simulink model "Explorer1632_dsPIC33EP512MU810_UART_Terminal_R2015b"  (R2015b)
settings: Solver=FixedStepDiscrete  StartTime=0.0  StopTime=inf  FixedStep=0.01  RelTol=1e-3
undefined symbols (not defined in the file): A0, D0, DiscIntNeverNeededParam, F4, F5, Max, ms, P100, P101, P16, P64, Pin, Resol, us
libraries: MCHP_Blockset x40, simulink x11
(part 2 of 2)

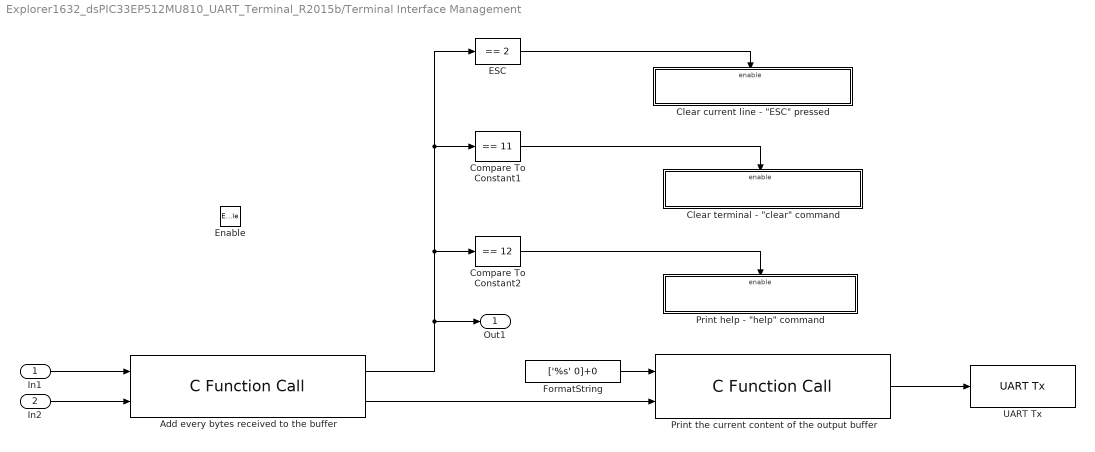
== system Explorer1632_dsPIC33EP512MU810_UART_Terminal_R2015b/Terminal Interface Management ==
  In1 : Inport
  In2 : Inport  Port=2
  Enable : EnablePort
  Add every bytes received to the buffer : MCHP_Blockset/User Functions/C Function Call  Priority=0  ParseFilesChkbx=off  ListFunctions1=Custom Function  Function1=unsigned char addToBuffer( unsigned char outputBuffer[100], unsigned char *rxBuffer, unsigned int rxCnt)  AddHeaderDeclaration=off  Function1Type=when block is updated (default)  Fct1BlockIn=rxBuffer, rxCnt  FctReturnBlockOut=on  Fct1BlockOut=outputBuffer  DataCollected=0  ORDERING=None  SampleTime=-1  S_INPUT="[2  5]"  S_INPUT_Size="[-1  0  0  0  0  0  0  0  0  0  0  0  0  0  0  0  0  0  0  0]"  S_OUTPUT=[2]  S_OUTPUT_Size="[1  17   0   0   0   0   0   0   0   0]"  S_ListCustomDatatype=S.S_ListCustomDatatype={};  MCHP_CRC=1191397  MCHP_MASTERLINK=Explorer1632_dsPIC33EP512MU810_UART_Terminal_R2015b/Explorer16//32 - dsPIC33EP512MU810/Microchip Master  PinDigitalInput=[]  PinDigitalOutput=[]  PinAnalogInput=[]
  "Clear current line - \"ESC\" pressed" : Subsystem  Priority=1  TreatAsAtomicUnit=on
  "Clear terminal - \"clear\" command" : Subsystem  Priority=100
  Compare To Constant1 : simulink/Logic and Bit Operations/Compare To Constant  relop===  const=11  OutDataTypeStr=uint8
  Compare To Constant2 : simulink/Logic and Bit Operations/Compare To Constant  relop===  const=12  OutDataTypeStr=uint8
  ESC : simulink/Logic and Bit Operations/Compare To Constant  relop===  const=2  OutDataTypeStr=uint8
  "FormatString " : Constant  Priority=15  Value=['%s' 0]+0  OutDataTypeStr=uint8  LockScale=on
  "Print help - \"help\" command" : Subsystem  Priority=99
  Print the current content of the output buffer : MCHP_Blockset/User Functions/C Function Call  Priority=16  ParseFilesChkbx=off  ListFunctions1=Custom Function  Function1=void sprintf(unsigned char outputBuffer[100], const unsigned char* formatString, unsigned char* rxBuffer)  AddHeaderDeclaration=off  Function1Type=when block is updated (default)  Fct1BlockIn=formatString , rxBuffer  FctReturnBlockOut=off  Fct1BlockOut=outputBuffer  DataCollected=0  ORDERING=None  SampleTime=-1  S_INPUT="[2  5]"  S_INPUT_Size="[-1  0  0  0  0  0  0  0  0  0  0  0  0  0  0  0  0  0  0  0]"  S_OUTPUT=[2]  S_OUTPUT_Size="[1  17   0   0   0   0   0   0   0   0]"  S_ListCustomDatatype=S.S_ListCustomDatatype={};  MCHP_CRC=1218869  MCHP_MASTERLINK=Explorer1632_dsPIC33EP512MU810_UART_Terminal_R2015b/Explorer16//32 - dsPIC33EP512MU810/Microchip Master  PinDigitalInput=[]  PinDigitalOutput=[]  PinAnalogInput=[]
  UART Tx : MCHP_Blockset/BUS UART/UART Tx  Priority=17  UART_REF=1  ORDERING=None  AllOrNothing=off  SampleTime=-1  MCHP_MASTERLINK=Explorer1632_dsPIC33EP512MU810_UART_Terminal_R2015b/Explorer16//32 - dsPIC33EP512MU810/Microchip Master  NSend_Input=off  UART_String=on  NSend_Output=off
  Out1 : Outport
  wires:
  In1/1 -> Add every bytes received to the buffer/1
  In2/1 -> Add every bytes received to the buffer/2
  "FormatString "/1 -> Print the current content of the output buffer/1
  Print the current content of the output buffer/1 -> UART Tx/1
  Add every bytes received to the buffer/2 -> Print the current content of the output buffer/2
  Add every bytes received to the buffer/1 -> Compare To Constant2/1, ESC/1, Compare To Constant1/1, Out1/1
  Compare To Constant1/1 -> "Clear terminal - \"clear\" command"/Enable
  Compare To Constant2/1 -> "Print help - \"help\" command"/Enable
  ESC/1 -> "Clear current line - \"ESC\" pressed"/Enable

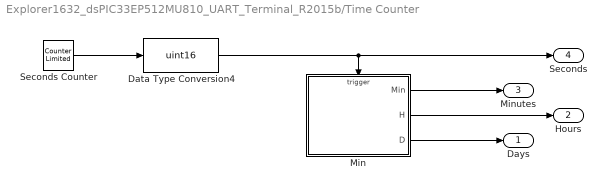
== system Explorer1632_dsPIC33EP512MU810_UART_Terminal_R2015b/Time Counter ==
  Data Type Conversion4 : DataTypeConversion  OutDataTypeStr=uint16  ConvertRealWorld=Stored Integer (SI)
  Min : Subsystem
  Seconds Counter : simulink/Sources/Counter Limited  uplimit=59  tsamp=1
  Days : Outport
  Hours : Outport  Port=2
  Minutes : Outport  Port=3
  Seconds : Outport  Port=4
  wires:
  Data Type Conversion4/1 -> Min/Trigger, Seconds/1
  Seconds Counter/1 -> Data Type Conversion4/1
  Min/1(Min) -> Minutes/1
  Min/2(H) -> Hours/1
  Min/3(D) -> Days/1

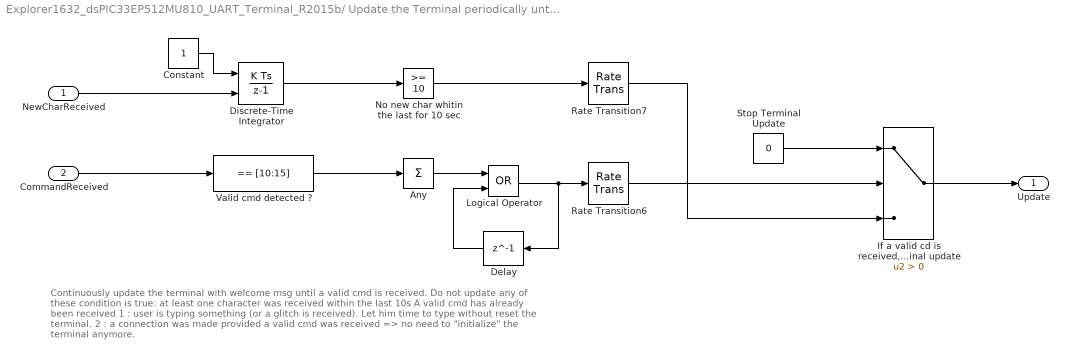
== system Explorer1632_dsPIC33EP512MU810_UART_Terminal_R2015b/ Update the Terminal periodically until a connection is detected /Periodic update until a valid cmd is received ==
  note: Continuously update the terminal with welcome msg until a valid cmd is received.
      |
      | Do not update any of these condition is true:
      | at least one character was received within the last 10s
      | A valid cmd has already been received
      |
      | 1 : user is typing something (or a glitch is received). Let him time to type without reset the terminal.
      | 2 : a connection was made provided a valid cmd was received => no need to "initialize" the terminal anymore.
  NewCharReceived : Inport
  CommandReceived : Inport  Port=2
  Any : Sum  Inputs=+
  Constant : Constant  OutDataTypeStr=uint16  SampleTime=.01
  Delay : Delay  DelayLength=1  InitialCondition=0
  Discrete-Time Integrator : DiscreteIntegrator  gainval=1  ExternalReset=level  InitialConditionSetting=State (most efficient)  SampleTime=-1  OutMax=[10]  OutDataTypeStr=fixdt(0,16)  SaturateOnIntegerOverflow=on  ICPrevOutput=DiscIntNeverNeededParam  ICPrevScaledInput=DiscIntNeverNeededParam
  "If a valid cd is received, then disable the trigger for terminal update" : Switch  Criteria=u2 > Threshold
  Logical Operator : Logic  Operator=OR  AllPortsSameDT=off  OutDataTypeStr=boolean
  No new char whitin the last for 10 sec : simulink/Logic and Bit Operations/Compare To Constant  relop=>=  const=10  OutDataTypeStr=boolean
  Rate Transition6 : RateTransition  Integrity=off  Deterministic=off  OutPortSampleTime=2
  Rate Transition7 : RateTransition  Integrity=off  Deterministic=off  OutPortSampleTime=2
  Stop Terminal Update : Constant  Value=0  OutDataTypeStr=uint16  SampleTime=-1
  Valid cmd detected ? : simulink/Logic and Bit Operations/Compare To Constant  relop===  const=[10:15]  OutDataTypeStr=boolean
  Update : Outport
  wires:
  NewCharReceived/1 -> Discrete-Time Integrator/2
  CommandReceived/1 -> Valid cmd detected ?/1
  Constant/1 -> Discrete-Time Integrator/1
  Valid cmd detected ?/1 -> Any/1
  Logical Operator/1 -> Delay/1, Rate Transition6/1
  Delay/1 -> Logical Operator/2
  Any/1 -> Logical Operator/1
  No new char whitin the last for 10 sec/1 -> Rate Transition7/1
  Discrete-Time Integrator/1 -> No new char whitin the last for 10 sec/1
  "If a valid cd is received, then disable the trigger for terminal update"/1 -> Update/1
  Stop Terminal Update/1 -> "If a valid cd is received, then disable the trigger for terminal update"/1
  Rate Transition6/1 -> "If a valid cd is received, then disable the trigger for terminal update"/2
  Rate Transition7/1 -> "If a valid cd is received, then disable the trigger for terminal update"/3

== system Explorer1632_dsPIC33EP512MU810_UART_Terminal_R2015b/ Update the Terminal periodically until a connection is detected /Periodic update until first character is received ==
  NewCharReceived : Inport
  Any char received? : simulink/Logic and Bit Operations/Compare To Constant  relop=>=  const=1  OutDataTypeStr=boolean
  Delay1 : Delay  DelayLength=1  InitialCondition=0
  Logical Operator : Logic  Operator=NOT  AllPortsSameDT=off  OutDataTypeStr=boolean
  Logical Operator1 : Logic  Operator=OR  AllPortsSameDT=off  OutDataTypeStr=boolean
  Rate Transition3 : RateTransition  Integrity=off  Deterministic=off  OutPortSampleTime=2
  Out1 : Outport
  wires:
  Any char received?/1 -> Logical Operator1/1
  NewCharReceived/1 -> Any char received?/1
  Rate Transition3/1 -> Out1/1
  Logical Operator/1 -> Rate Transition3/1
  Delay1/1 -> Logical Operator1/2
  Logical Operator1/1 -> Logical Operator/1, Delay1/1

== system Explorer1632_dsPIC33EP512MU810_UART_Terminal_R2015b/ Update the Terminal periodically until a connection is detected /Terminal Initialization ==
  note: Re-initialize the terminal and display the main menu every 2 second until a valid cmd is received. This allows initializing hot plugged terminal.
  note: => command to r eset the terminal to initial state:
      | Go home and then set green color for text
  Enable : EnablePort
  Constant7 : Constant  Priority=0  Value="[27 99  0]+0"  OutDataTypeStr=int8  LockScale=on
  "Print help - \"help\" command" : Subsystem  Priority=99
  UART Tx1 : MCHP_Blockset/BUS UART/UART Tx  UART_REF=1  ORDERING=None  AllOrNothing=off  SampleTime=-1  MCHP_MASTERLINK=Explorer1632_dsPIC33EP512MU810_UART_Terminal_R2015b/Explorer16//32 - dsPIC33EP512MU810/Microchip Master  NSend_Input=off  UART_String=on  NSend_Output=off
  wires:
  Constant7/1 -> UART Tx1/1

== system Explorer1632_dsPIC33EP512MU810_UART_Terminal_R2015b/Data Collector/Temperature Calibration  ==
  Temp raw : Inport
  "100 deg / Volt " : Gain  Gain=3.3/(2^16) * 100  OutDataTypeStr=single
  Calibration Offset 500 mv at 0 deg : Constant  Value=50  OutDataTypeStr=Inherit: Inherit via back propagation  SampleTime=-1
  Sum2 : Sum  Inputs=|+-  OutDataTypeStr=Inherit: Same as first input
  Temp degC : Outport
  wires:
  Temp raw/1 -> "100 deg / Volt "/1
  "100 deg / Volt "/1 -> Sum2/1
  Calibration Offset 500 mv at 0 deg/1 -> Sum2/2
  Sum2/1 -> Temp degC/1  "deg"

== system Explorer1632_dsPIC33EP512MU810_UART_Terminal_R2015b/Explorer16//32 - dsPIC33EP512MU810/Open board Documentation ==

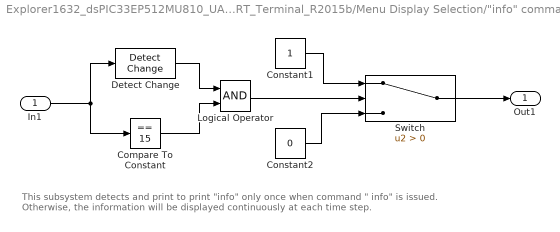
== system Explorer1632_dsPIC33EP512MU810_UART_Terminal_R2015b/Menu Display Selection/"info" command detection ==
  note: This subsystem detects and print to print "info" only once when command " info" is issued. Otherwise, the information will be displayed continuously at each time step.
  In1 : Inport
  Compare To Constant : simulink/Logic and Bit Operations/Compare To Constant  relop===  const=15  OutDataTypeStr=uint8
  Constant1 : Constant  OutDataTypeStr=uint16
  Constant2 : Constant  Value=0  OutDataTypeStr=uint16
  Detect Change : simulink/Logic and Bit Operations/Detect Change  vinit=0  OutDataTypeStr=boolean
  Logical Operator : Logic  AllPortsSameDT=off  OutDataTypeStr=boolean
  Switch : Switch  Criteria=u2 > Threshold
  Out1 : Outport
  wires:
  Constant2/1 -> Switch/3
  Constant1/1 -> Switch/1
  Switch/1 -> Out1/1
  Compare To Constant/1 -> Logical Operator/2
  Logical Operator/1 -> Switch/2
  Detect Change/1 -> Logical Operator/1
  In1/1 -> Detect Change/1, Compare To Constant/1

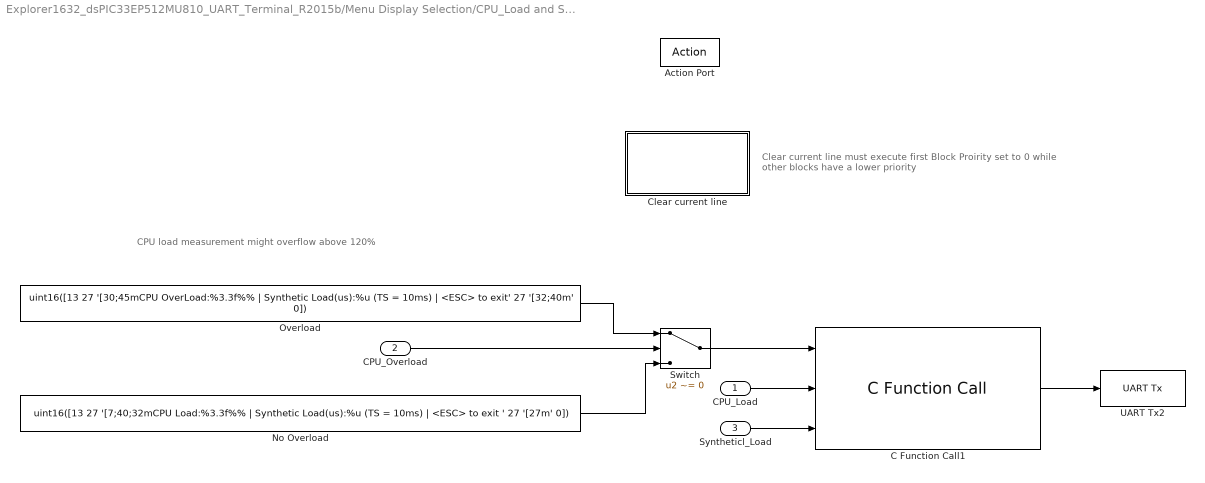
== system Explorer1632_dsPIC33EP512MU810_UART_Terminal_R2015b/Menu Display Selection/CPU_Load and Synthetic_Load ==
  note: Clear current line must execute first
      | Block Proirity set to 0 while other blocks have a lower priority
  note: CPU load measurement might overflow above 120%
  CPU_Load : Inport
  CPU_Overload : Inport  Port=2
  Syntheticl_Load : Inport  Port=3
  Action Port : ActionPort  ActionType=case
  C Function Call1 : MCHP_Blockset/User Functions/C Function Call  Priority=20  ParseFilesChkbx=off  ListFunctions1=Custom Function  Function1=void sprintf(char outputBuffer[100], const char* formatString, float arg1, unsigned int arg2)  AddHeaderDeclaration=off  Function1Type=when block is updated (default)  Fct1BlockIn=formatString , arg1, arg2  FctReturnBlockOut=off  Fct1BlockOut=outputBuffer  DataCollected=0  ORDERING=None  SampleTime=-1  S_INPUT="[2  5]"  S_INPUT_Size="[-1  0  0  0  0  0  0  0  0  0  0  0  0  0  0  0  0  0  0  0]"  S_OUTPUT=[2]  S_OUTPUT_Size="[1  17   0   0   0   0   0   0   0   0]"  S_ListCustomDatatype=S.S_ListCustomDatatype={};  MCHP_CRC=1179584  MCHP_MASTERLINK=Explorer1632_dsPIC33EP512MU810_UART_Terminal_R2015b/Explorer16//32 - dsPIC33EP512MU810/Microchip Master  PinDigitalInput=[]  PinDigitalOutput=[]  PinAnalogInput=[]
  Clear current line : Subsystem  Priority=0  TreatAsAtomicUnit=on
  No Overload : Constant  Value="uint16([13 27 '[7;40;32mCPU Load:%3.3f%% |  Synthetic Load(us):%u (TS = 10ms) | <ESC> to exit     ' 27 '[27m'  0])"  OutDataTypeStr=int8  LockScale=on
  Overload : Constant  Value="uint16([13 27 '[30;45mCPU OverLoad:%3.3f%% |  Synthetic Load(us):%u (TS = 10ms) | <ESC> to exit' 27 '[32;40m'  0])"  OutDataTypeStr=int8  LockScale=on
  Switch : Switch  Criteria=u2 ~= 0
  UART Tx2 : MCHP_Blockset/BUS UART/UART Tx  UART_REF=1  ORDERING=None  AllOrNothing=off  SampleTime=-1  MCHP_MASTERLINK=Explorer1632_dsPIC33EP512MU810_UART_Terminal_R2015b/Explorer16//32 - dsPIC33EP512MU810/Microchip Master  NSend_Input=off  UART_String=on  NSend_Output=off
  wires:
  C Function Call1/1 -> UART Tx2/1
  CPU_Load/1 -> C Function Call1/2
  Syntheticl_Load/1 -> C Function Call1/3
  CPU_Overload/1 -> Switch/2
  Switch/1 -> C Function Call1/1
  No Overload/1 -> Switch/3
  Overload/1 -> Switch/1

== system Explorer1632_dsPIC33EP512MU810_UART_Terminal_R2015b/Menu Display Selection/Info ==
  In1 : Inport
  Action Port : ActionPort  ActionType=case
  "Print \"info\"" : Subsystem
  wires:
  In1/1 -> "Print \"info\""/Enable

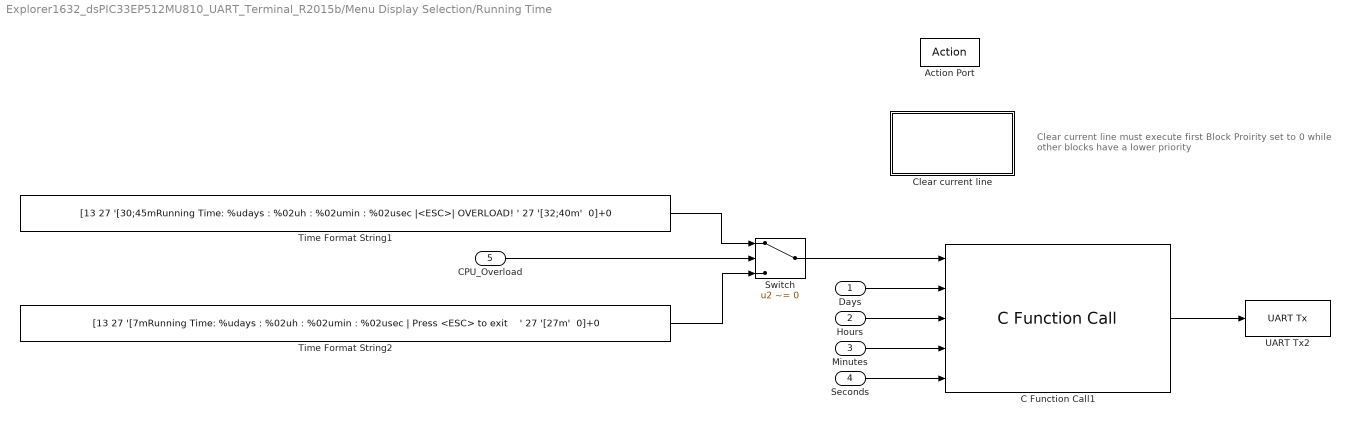
== system Explorer1632_dsPIC33EP512MU810_UART_Terminal_R2015b/Menu Display Selection/Running Time ==
  note: Clear current line must execute first
      | Block Proirity set to 0 while other blocks have a lower priority
  Days : Inport
  Hours : Inport  Port=2
  Minutes : Inport  Port=3
  Seconds : Inport  Port=4
  CPU_Overload : Inport  Port=5
  Action Port : ActionPort  ActionType=case
  C Function Call1 : MCHP_Blockset/User Functions/C Function Call  ParseFilesChkbx=off  ListFunctions1=Custom Function  Function1=void sprintf(char outputBuffer[100], const char* formatString, unsigned int days,unsigned int hours,unsigned int minutes,unsigned int seconds)  AddHeaderDeclaration=off  Function1Type=when block is updated (default)  Fct1BlockIn=formatString, days, , hours, minutes, seconds  FctReturnBlockOut=off  Fct1BlockOut=outputBuffer  DataCollected=0  ORDERING=None  SampleTime=-1  S_INPUT="[2  5]"  S_INPUT_Size="[-1  0  0  0  0  0  0  0  0  0  0  0  0  0  0  0  0  0  0  0]"  S_OUTPUT=[2]  S_OUTPUT_Size="[1  17   0   0   0   0   0   0   0   0]"  S_ListCustomDatatype=S.S_ListCustomDatatype={};  MCHP_CRC=1463372  MCHP_MASTERLINK=Explorer1632_dsPIC33EP512MU810_UART_Terminal_R2015b/Explorer16//32 - dsPIC33EP512MU810/Microchip Master  PinDigitalInput=[]  PinDigitalOutput=[]  PinAnalogInput=[]
  Clear current line : Subsystem  Priority=0  TreatAsAtomicUnit=on
  Switch : Switch  Criteria=u2 ~= 0
  Time Format String1 : Constant  Value="[13 27 '[30;45mRunning Time: %udays : %02uh : %02umin : %02usec |<ESC>| OVERLOAD! ' 27 '[32;40m'  0]+0"  OutDataTypeStr=int8  LockScale=on
  Time Format String2 : Constant  Value="[13 27 '[7mRunning Time: %udays : %02uh : %02umin : %02usec | Press <ESC> to exit    ' 27 '[27m'  0]+0"  OutDataTypeStr=int8  LockScale=on
  UART Tx2 : MCHP_Blockset/BUS UART/UART Tx  UART_REF=1  ORDERING=None  AllOrNothing=off  SampleTime=-1  MCHP_MASTERLINK=Explorer1632_dsPIC33EP512MU810_UART_Terminal_R2015b/Explorer16//32 - dsPIC33EP512MU810/Microchip Master  NSend_Input=off  UART_String=on  NSend_Output=off
  wires:
  C Function Call1/1 -> UART Tx2/1
  Switch/1 -> C Function Call1/1
  Minutes/1 -> C Function Call1/4
  Hours/1 -> C Function Call1/3
  Seconds/1 -> C Function Call1/5
  Days/1 -> C Function Call1/2
  Time Format String1/1 -> Switch/1
  Time Format String2/1 -> Switch/3
  CPU_Overload/1 -> Switch/2

== system Explorer1632_dsPIC33EP512MU810_UART_Terminal_R2015b/Menu Display Selection/Temperature ==
  note: Clear current line must execute first
      | Block Proirity set to 0 while other blocks have a lower priority
  Temperature : Inport
  Action Port : ActionPort  ActionType=case
  C Function Call1 : MCHP_Blockset/User Functions/C Function Call  ParseFilesChkbx=off  ListFunctions1=Custom Function  Function1=void sprintf(char outputBuffer[100], const char* formatString, float temperature)  AddHeaderDeclaration=off  Function1Type=when block is updated (default)  Fct1BlockIn=formatString , temperature  FctReturnBlockOut=off  Fct1BlockOut=outputBuffer  DataCollected=0  ORDERING=None  SampleTime=-1  S_INPUT="[2  5]"  S_INPUT_Size="[-1  0  0  0  0  0  0  0  0  0  0  0  0  0  0  0  0  0  0  0]"  S_OUTPUT=[2]  S_OUTPUT_Size="[1  17   0   0   0   0   0   0   0   0]"  S_ListCustomDatatype=S.S_ListCustomDatatype={};  MCHP_CRC=1214402  MCHP_MASTERLINK=Explorer1632_dsPIC33EP512MU810_UART_Terminal_R2015b/Explorer16//32 - dsPIC33EP512MU810/Microchip Master  PinDigitalInput=[]  PinDigitalOutput=[]  PinAnalogInput=[]
  Clear current line : Subsystem  Priority=0  TreatAsAtomicUnit=on
  Temperature_FormatString : Constant  Value="[13 27 '[7m Temperature: %3.3f *C  Press <ESC> to exit' 27 '[27m'  0]+0"  OutDataTypeStr=int8  LockScale=on
  UART Tx2 : MCHP_Blockset/BUS UART/UART Tx  UART_REF=1  ORDERING=None  AllOrNothing=off  SampleTime=-1  MCHP_MASTERLINK=Explorer1632_dsPIC33EP512MU810_UART_Terminal_R2015b/Explorer16//32 - dsPIC33EP512MU810/Microchip Master  NSend_Input=off  UART_String=on  NSend_Output=off
  wires:
  C Function Call1/1 -> UART Tx2/1
  Temperature/1 -> C Function Call1/2
  Temperature_FormatString/1 -> C Function Call1/1

== system Explorer1632_dsPIC33EP512MU810_UART_Terminal_R2015b/Terminal Interface Management/Clear current line - "ESC" pressed ==
  Enable : EnablePort
  Clear current line : Subsystem  Priority=0  TreatAsAtomicUnit=on

== system Explorer1632_dsPIC33EP512MU810_UART_Terminal_R2015b/Terminal Interface Management/Clear terminal - "clear" command ==
  note: => command to r eset the terminal to initial state
  note: => Command for terminal to clear the entire screen. Set cursor to home
  Enable : EnablePort
  Mux : Mux  Inputs=3
  Reset terminal : Constant  Priority=0  Value=uint8([27 '[2J'])  LockScale=on
  Set cursor home : Constant  Priority=0  Value=uint8([27 '[H'])  LockScale=on
  UART Tx1 Send all : MCHP_Blockset/BUS UART/UART Tx  UART_REF=1  ORDERING=None  AllOrNothing=off  SampleTime=-1  MCHP_MASTERLINK=Explorer1632_dsPIC33EP512MU810_UART_Terminal_R2015b/Explorer16//32 - dsPIC33EP512MU810/Microchip Master  NSend_Input=off  UART_String=off  NSend_Output=off
  termination : Constant  Priority=0  Value=uint8(0)  LockScale=on
  wires:
  Reset terminal/1 -> Mux/1
  Set cursor home/1 -> Mux/2
  Mux/1 -> UART Tx1 Send all/1
  termination/1 -> Mux/3

== system Explorer1632_dsPIC33EP512MU810_UART_Terminal_R2015b/Terminal Interface Management/Print help - "help" command ==
  note: => print help info
  Enable : EnablePort
  Help C Function Call : MCHP_Blockset/User Functions/C Function Call  Priority=0  ParseFilesChkbx=off  ListFunctions1=Custom Function  Function1=void printHelp(unsigned char str[5000])  AddHeaderDeclaration=off  Function1Type=when block is updated (default)  FctReturnBlockOut=off  Fct1BlockOut=str  DataCollected=0  ORDERING=None  SampleTime=-1  S_INPUT="[2  5]"  S_INPUT_Size="[-1  0  0  0  0  0  0  0  0  0  0  0  0  0  0  0  0  0  0  0]"  S_OUTPUT=[2]  S_OUTPUT_Size="[1  17   0   0   0   0   0   0   0   0]"  S_ListCustomDatatype=S.S_ListCustomDatatype={};  MCHP_CRC=867293  MCHP_MASTERLINK=Explorer1632_dsPIC33EP512MU810_UART_Terminal_R2015b/Explorer16//32 - dsPIC33EP512MU810/Microchip Master  PinDigitalInput=[]  PinDigitalOutput=[]  PinAnalogInput=[]
  UART Tx2 : MCHP_Blockset/BUS UART/UART Tx  UART_REF=1  ORDERING=None  AllOrNothing=off  SampleTime=-1  MCHP_MASTERLINK=Explorer1632_dsPIC33EP512MU810_UART_Terminal_R2015b/Explorer16//32 - dsPIC33EP512MU810/Microchip Master  NSend_Input=off  UART_String=on  NSend_Output=off
  wires:
  Help C Function Call/1 -> UART Tx2/1

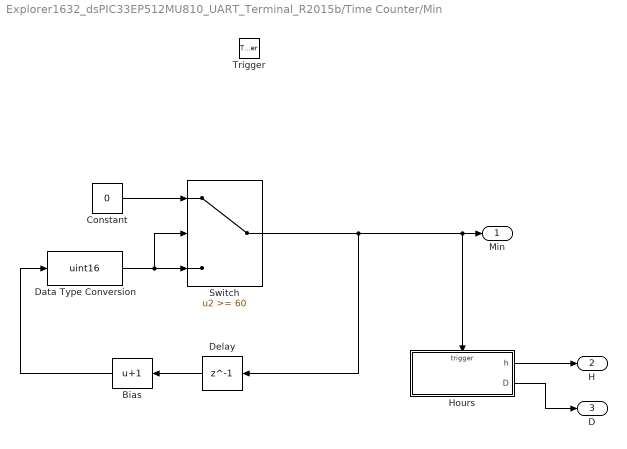
== system Explorer1632_dsPIC33EP512MU810_UART_Terminal_R2015b/Time Counter/Min ==
  Trigger : TriggerPort  TriggerType=falling  PortDimensions=1
  Bias : Bias  Bias=1
  Constant : Constant  Value=0  OutDataTypeStr=uint16
  Data Type Conversion : DataTypeConversion  OutDataTypeStr=uint16
  Delay : Delay  DelayLength=1  InitialCondition=0
  Hours : Subsystem
  Switch : Switch  Threshold=60
  Min : Outport
  H : Outport  Port=2
  D : Outport  Port=3
  wires:
  Constant/1 -> Switch/1
  Switch/1 -> Hours/Trigger, Min/1, Delay/1
  Delay/1 -> Bias/1
  Bias/1 -> Data Type Conversion/1
  Data Type Conversion/1 -> Switch/2, Switch/3
  Hours/1(h) -> H/1
  Hours/2(D) -> D/1

== system Explorer1632_dsPIC33EP512MU810_UART_Terminal_R2015b/ Update the Terminal periodically until a connection is detected /Terminal Initialization/Print help - "help" command ==
  note: => print help info
  Help C Function Call : MCHP_Blockset/User Functions/C Function Call  Priority=0  ParseFilesChkbx=off  ListFunctions1=Custom Function  Function1=void printHelp(unsigned char str[1500])  AddHeaderDeclaration=off  Function1Type=when block is updated (default)  FctReturnBlockOut=off  Fct1BlockOut=str  DataCollected=0  ORDERING=None  SampleTime=-1  S_INPUT="[2  5]"  S_INPUT_Size="[-1  0  0  0  0  0  0  0  0  0  0  0  0  0  0  0  0  0  0  0]"  S_OUTPUT=[2]  S_OUTPUT_Size="[1  17   0   0   0   0   0   0   0   0]"  S_ListCustomDatatype=S.S_ListCustomDatatype={};  MCHP_CRC=867001  MCHP_MASTERLINK=Explorer1632_dsPIC33EP512MU810_UART_Terminal_R2015b/Explorer16//32 - dsPIC33EP512MU810/Microchip Master  PinDigitalInput=[]  PinDigitalOutput=[]  PinAnalogInput=[]
  UART Tx2 : MCHP_Blockset/BUS UART/UART Tx  UART_REF=1  ORDERING=None  AllOrNothing=off  SampleTime=-1  MCHP_MASTERLINK=Explorer1632_dsPIC33EP512MU810_UART_Terminal_R2015b/Explorer16//32 - dsPIC33EP512MU810/Microchip Master  NSend_Input=off  UART_String=on  NSend_Output=off
  wires:
  Help C Function Call/1 -> UART Tx2/1

== system Explorer1632_dsPIC33EP512MU810_UART_Terminal_R2015b/Menu Display Selection/CPU_Load and Synthetic_Load/Clear current line ==
  C Function Call2 : MCHP_Blockset/User Functions/C Function Call  ParseFilesChkbx=off  ListFunctions1=Custom Function  Function1=void sprintf(unsigned char outputBuffer[100], const unsigned char* formatString)  AddHeaderDeclaration=off  Function1Type=when block is updated (default)  Fct1BlockIn=formatString  FctReturnBlockOut=off  Fct1BlockOut=outputBuffer  DataCollected=0  ORDERING=None  SampleTime=-1  S_INPUT="[2  5]"  S_INPUT_Size="[-1  0  0  0  0  0  0  0  0  0  0  0  0  0  0  0  0  0  0  0]"  S_OUTPUT=[2]  S_OUTPUT_Size="[1  17   0   0   0   0   0   0   0   0]"  S_ListCustomDatatype=S.S_ListCustomDatatype={};  MCHP_CRC=1122806  MCHP_MASTERLINK=Explorer1632_dsPIC33EP512MU810_UART_Terminal_R2015b/Explorer16//32 - dsPIC33EP512MU810/Microchip Master  PinDigitalInput=[]  PinDigitalOutput=[]  PinAnalogInput=[]
  Constant1 : Constant  Value=[13 27 '[2K' 0]+0  OutDataTypeStr=uint8  LockScale=on
  UART Tx1 : MCHP_Blockset/BUS UART/UART Tx  UART_REF=1  ORDERING=None  AllOrNothing=off  SampleTime=-1  MCHP_MASTERLINK=Explorer1632_dsPIC33EP512MU810_UART_Terminal_R2015b/Explorer16//32 - dsPIC33EP512MU810/Microchip Master  NSend_Input=off  UART_String=on  NSend_Output=off
  wires:
  Constant1/1 -> C Function Call2/1
  C Function Call2/1 -> UART Tx1/1

== system Explorer1632_dsPIC33EP512MU810_UART_Terminal_R2015b/Menu Display Selection/Info/Print "info" ==
  Enable : EnablePort
  " Format String" : Constant  Value=['%s' 0]+0  OutDataTypeStr=int8  LockScale=on
  C Function Call1 : MCHP_Blockset/User Functions/C Function Call  ParseFilesChkbx=off  ListFunctions1=Custom Function  Function1=void sprintf(char outputBuffer[1500], const char* formatString, const unsigned char* info)  AddHeaderDeclaration=off  Function1Type=when block is updated (default)  Fct1BlockIn=formatString, info  FctReturnBlockOut=off  Fct1BlockOut=outputBuffer  DataCollected=0  ORDERING=None  SampleTime=-1  S_INPUT="[2  5]"  S_INPUT_Size="[-1  0  0  0  0  0  0  0  0  0  0  0  0  0  0  0  0  0  0  0]"  S_OUTPUT=[2]  S_OUTPUT_Size="[1  17   0   0   0   0   0   0   0   0]"  S_ListCustomDatatype=S.S_ListCustomDatatype={};  MCHP_CRC=1161349  MCHP_MASTERLINK=Explorer1632_dsPIC33EP512MU810_UART_Terminal_R2015b/Explorer16//32 - dsPIC33EP512MU810/Microchip Master  PinDigitalInput=[]  PinDigitalOutput=[]  PinAnalogInput=[]
  C Function Call2 : MCHP_Blockset/User Functions/C Function Call  ParseFilesChkbx=off  ListFunctions1=Custom Function  Function1=void printInfo(unsigned char str[1500])  AddHeaderDeclaration=off  Function1Type=when block is updated (default)  FctReturnBlockOut=off  Fct1BlockOut=str  DataCollected=0  ORDERING=None  SampleTime=-1  S_INPUT="[2  5]"  S_INPUT_Size="[-1  0  0  0  0  0  0  0  0  0  0  0  0  0  0  0  0  0  0  0]"  S_OUTPUT=[2]  S_OUTPUT_Size="[1  17   0   0   0   0   0   0   0   0]"  S_ListCustomDatatype=S.S_ListCustomDatatype={};  MCHP_CRC=867296  MCHP_MASTERLINK=Explorer1632_dsPIC33EP512MU810_UART_Terminal_R2015b/Explorer16//32 - dsPIC33EP512MU810/Microchip Master  PinDigitalInput=[]  PinDigitalOutput=[]  PinAnalogInput=[]
  UART Tx2 : MCHP_Blockset/BUS UART/UART Tx  UART_REF=1  ORDERING=None  AllOrNothing=off  SampleTime=-1  MCHP_MASTERLINK=Explorer1632_dsPIC33EP512MU810_UART_Terminal_R2015b/Explorer16//32 - dsPIC33EP512MU810/Microchip Master  NSend_Input=off  UART_String=on  NSend_Output=off
  wires:
  " Format String"/1 -> C Function Call1/1
  C Function Call1/1 -> UART Tx2/1
  C Function Call2/1 -> C Function Call1/2

== system Explorer1632_dsPIC33EP512MU810_UART_Terminal_R2015b/Menu Display Selection/Running Time/Clear current line ==
  C Function Call2 : MCHP_Blockset/User Functions/C Function Call  ParseFilesChkbx=off  ListFunctions1=Custom Function  Function1=void sprintf(unsigned char outputBuffer[100], const unsigned char* formatString)  AddHeaderDeclaration=off  Function1Type=when block is updated (default)  Fct1BlockIn=formatString  FctReturnBlockOut=off  Fct1BlockOut=outputBuffer  DataCollected=0  ORDERING=None  SampleTime=-1  S_INPUT="[2  5]"  S_INPUT_Size="[-1  0  0  0  0  0  0  0  0  0  0  0  0  0  0  0  0  0  0  0]"  S_OUTPUT=[2]  S_OUTPUT_Size="[1  17   0   0   0   0   0   0   0   0]"  S_ListCustomDatatype=S.S_ListCustomDatatype={};  MCHP_CRC=1122806  MCHP_MASTERLINK=Explorer1632_dsPIC33EP512MU810_UART_Terminal_R2015b/Explorer16//32 - dsPIC33EP512MU810/Microchip Master  PinDigitalInput=[]  PinDigitalOutput=[]  PinAnalogInput=[]
  Constant1 : Constant  Value=[13 27 '[2K' 0]+0  OutDataTypeStr=uint8  LockScale=on
  UART Tx1 : MCHP_Blockset/BUS UART/UART Tx  UART_REF=1  ORDERING=None  AllOrNothing=off  SampleTime=-1  MCHP_MASTERLINK=Explorer1632_dsPIC33EP512MU810_UART_Terminal_R2015b/Explorer16//32 - dsPIC33EP512MU810/Microchip Master  NSend_Input=off  UART_String=on  NSend_Output=off
  wires:
  C Function Call2/1 -> UART Tx1/1
  Constant1/1 -> C Function Call2/1

== system Explorer1632_dsPIC33EP512MU810_UART_Terminal_R2015b/Menu Display Selection/Temperature/Clear current line ==
  C Function Call2 : MCHP_Blockset/User Functions/C Function Call  ParseFilesChkbx=off  ListFunctions1=Custom Function  Function1=void sprintf(unsigned char outputBuffer[100], const unsigned char* formatString)  AddHeaderDeclaration=off  Function1Type=when block is updated (default)  Fct1BlockIn=formatString  FctReturnBlockOut=off  Fct1BlockOut=outputBuffer  DataCollected=0  ORDERING=None  SampleTime=-1  S_INPUT="[2  5]"  S_INPUT_Size="[-1  0  0  0  0  0  0  0  0  0  0  0  0  0  0  0  0  0  0  0]"  S_OUTPUT=[2]  S_OUTPUT_Size="[1  17   0   0   0   0   0   0   0   0]"  S_ListCustomDatatype=S.S_ListCustomDatatype={};  MCHP_CRC=1122806  MCHP_MASTERLINK=Explorer1632_dsPIC33EP512MU810_UART_Terminal_R2015b/Explorer16//32 - dsPIC33EP512MU810/Microchip Master  PinDigitalInput=[]  PinDigitalOutput=[]  PinAnalogInput=[]
  Constant1 : Constant  Value=[13 27 '[2K' 0]+0  OutDataTypeStr=uint8  LockScale=on
  UART Tx1 : MCHP_Blockset/BUS UART/UART Tx  UART_REF=1  ORDERING=None  AllOrNothing=off  SampleTime=-1  MCHP_MASTERLINK=Explorer1632_dsPIC33EP512MU810_UART_Terminal_R2015b/Explorer16//32 - dsPIC33EP512MU810/Microchip Master  NSend_Input=off  UART_String=on  NSend_Output=off
  wires:
  C Function Call2/1 -> UART Tx1/1
  Constant1/1 -> C Function Call2/1

== system Explorer1632_dsPIC33EP512MU810_UART_Terminal_R2015b/Terminal Interface Management/Clear current line - "ESC" pressed/Clear current line ==
  C Function Call2 : MCHP_Blockset/User Functions/C Function Call  ParseFilesChkbx=off  ListFunctions1=Custom Function  Function1=void sprintf(unsigned char outputBuffer[100], const unsigned char* formatString)  AddHeaderDeclaration=off  Function1Type=when block is updated (default)  Fct1BlockIn=formatString  FctReturnBlockOut=off  Fct1BlockOut=outputBuffer  DataCollected=0  ORDERING=None  SampleTime=-1  S_INPUT="[2  5]"  S_INPUT_Size="[-1  0  0  0  0  0  0  0  0  0  0  0  0  0  0  0  0  0  0  0]"  S_OUTPUT=[2]  S_OUTPUT_Size="[1  17   0   0   0   0   0   0   0   0]"  S_ListCustomDatatype=S.S_ListCustomDatatype={};  MCHP_CRC=1122806  MCHP_MASTERLINK=Explorer1632_dsPIC33EP512MU810_UART_Terminal_R2015b/Explorer16//32 - dsPIC33EP512MU810/Microchip Master  PinDigitalInput=[]  PinDigitalOutput=[]  PinAnalogInput=[]
  Constant1 : Constant  Value=uint8([13 27 '[2K' 0])  OutDataTypeStr=uint8  LockScale=on
  UART Tx1 : MCHP_Blockset/BUS UART/UART Tx  UART_REF=1  ORDERING=None  AllOrNothing=off  SampleTime=-1  MCHP_MASTERLINK=Explorer1632_dsPIC33EP512MU810_UART_Terminal_R2015b/Explorer16//32 - dsPIC33EP512MU810/Microchip Master  NSend_Input=off  UART_String=on  NSend_Output=off
  wires:
  Constant1/1 -> C Function Call2/1
  C Function Call2/1 -> UART Tx1/1

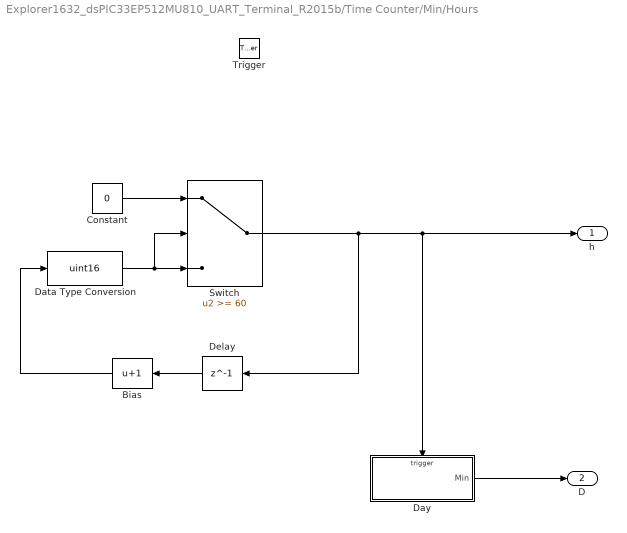
== system Explorer1632_dsPIC33EP512MU810_UART_Terminal_R2015b/Time Counter/Min/Hours ==
  Trigger : TriggerPort  TriggerType=falling  PortDimensions=1
  Bias : Bias  Bias=1
  Constant : Constant  Value=0  OutDataTypeStr=uint16
  Data Type Conversion : DataTypeConversion  OutDataTypeStr=uint16
  Day : Subsystem
  Delay : Delay  DelayLength=1  InitialCondition=0
  Switch : Switch  Threshold=60
  h : Outport
  D : Outport  Port=2
  wires:
  Constant/1 -> Switch/1
  Switch/1 -> h/1, Day/Trigger, Delay/1
  Delay/1 -> Bias/1
  Bias/1 -> Data Type Conversion/1
  Data Type Conversion/1 -> Switch/2, Switch/3
  Day/1(Min) -> D/1

== system Explorer1632_dsPIC33EP512MU810_UART_Terminal_R2015b/Time Counter/Min/Hours/Day ==
  Trigger : TriggerPort  TriggerType=falling  PortDimensions=1
  Bias : Bias  Bias=1
  Constant : Constant  Value=0  OutDataTypeStr=uint16
  Data Type Conversion : DataTypeConversion  OutDataTypeStr=uint16
  Delay : Delay  DelayLength=1  InitialCondition=0
  Switch : Switch  Threshold=60
  Min : Outport
  wires:
  Constant/1 -> Switch/1
  Switch/1 -> Min/1, Delay/1
  Delay/1 -> Bias/1
  Bias/1 -> Data Type Conversion/1
  Data Type Conversion/1 -> Switch/2, Switch/3
